simulink model "joint_space_pd_w_g_comp"  (R2021b)
settings: Solver=FixedStepAuto  StartTime=0.0  StopTime=2  FixedStep=Ts  RelTol=1e-3
undefined symbols (not defined in the file): addNoise, dqi, g_q, KD, KP, myRobot, qd, qi
libraries: vrlib x1
settings Model: Creator=simon  LastModifiedBy=luigi
settings SolverCC: ZeroCrossControl=DisableAll  AlgebraicLoopSolver=TrustRegion
settings DebuggingCC: SFMachineParentedDataDiag=warning

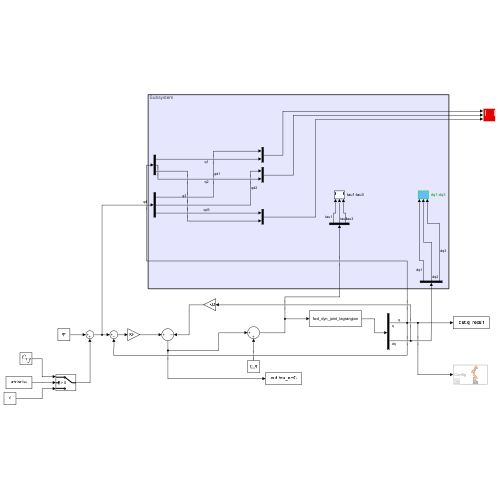
[thumbnail: Simulink's stored preview of the top-level diagram]
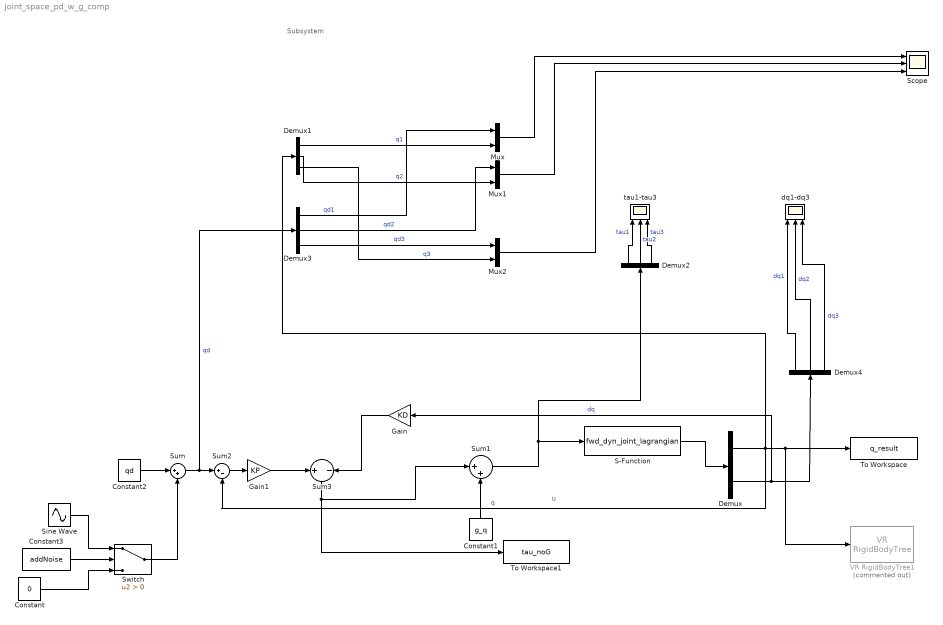
== system joint_space_pd_w_g_comp ==
  note: Subsystem
  note: u
  Constant : Constant  Value=0
  Constant1 : Constant  Value=g_q
  Constant2 : Constant  Value=qd
  Constant3 : Constant  Value=addNoise
  Demux : Demux  Outputs=2
  Demux{1..4} (4 alike) : Demux  Outputs=myRobot.N
  Gain : Gain  Gain=KD
  Gain1 : Gain  Gain=KP
  Mux : Mux  Inputs=2
  Mux1 : Mux  Inputs=2
  Mux2 : Mux  Inputs=2
  S-Function : S-Function  FunctionName=fwd_dyn_joint_lagrangian  Parameters=myRobot,qi,dqi  SFunctionDeploymentMode=off  EnableBusSupport=off
  Scope : Scope  NumInputPorts=3
  Sine Wave : Sin  Amplitude=0.1  Frequency=5  SampleTime=0
  Sum : Sum  Inputs=|++
  Sum1 : Sum  Inputs=|++
  Sum2 : Sum  Inputs=|+-
  Sum3 : Sum  Inputs=+||-
  Switch : Switch  Criteria=u2 > Threshold
  To Workspace : ToWorkspace  VariableName=q_result  SaveFormat=Timeseries  SampleTime=-1
  To Workspace1 : ToWorkspace  VariableName=tau_noG  SaveFormat=Timeseries  SampleTime=-1
  VR RigidBodyTree1 : vrlib/VR RigidBodyTree  Commented=on  RBT=rbt  useRBT=on  Ts=-1  ForceViewerOpen=on
      settings: SourceProductBaseCode=SL
  dq1-dq3 : Scope  NumInputPorts=3
  tau1-tau3 : Scope  NumInputPorts=3
  wires:
  Demux/1 -> VR RigidBodyTree1/1, To Workspace/1, Demux1/1, Sum2/2  "q"
  Sum3/1 -> To Workspace1/1, Sum1/1
  S-Function/1 -> Demux/1
  Demux/2 -> Demux4/1, Gain/1  "dq"
  Sum2/1 -> Gain1/1
  Gain1/1 -> Sum3/1
  Gain/1 -> Sum3/2
  Constant2/1 -> Sum/1
  Constant/1 -> Switch/3
  Sine Wave/1 -> Switch/1
  Sum/1 -> Demux3/1, Sum2/1  "qd"
  Switch/1 -> Sum/2
  Constant1/1 -> Sum1/2
  Constant3/1 -> Switch/2
  Sum1/1 -> Demux2/1, S-Function/1
  Mux2/1 -> Scope/3
  Demux3/3 -> Mux2/1  "qd3"
  Demux1/2 -> Mux1/2  "q2"
  Demux4/3 -> dq1-dq3/3  "dq3"
  Demux4/2 -> dq1-dq3/2  "dq2"
  Demux4/1 -> dq1-dq3/1  "dq1"
  Mux1/1 -> Scope/2
  Demux2/1 -> tau1-tau3/1  "tau1"
  Demux2/2 -> tau1-tau3/2  "tau2"
  Demux3/1 -> Mux/1  "qd1"
  Demux2/3 -> tau1-tau3/3  "tau3"
  Mux/1 -> Scope/1
  Demux1/1 -> Mux/2  "q1"
  Demux3/2 -> Mux1/1  "qd2"
  Demux1/3 -> Mux2/2  "q3"
